simulink model "c00010M_harness"  (R2018a)
settings: Solver=FixedStepAuto  StartTime=0.0  StopTime=300  FixedStep=0.1  RelTol=1e-3
undefined symbols (not defined in the file): A1, hmax, PriorityTank, R1, R2, sigbuilder_block, TempThreshold
(part 1 of 40)
settings Model: Creator=aarrieta  LastModifiedBy=umarkiegi

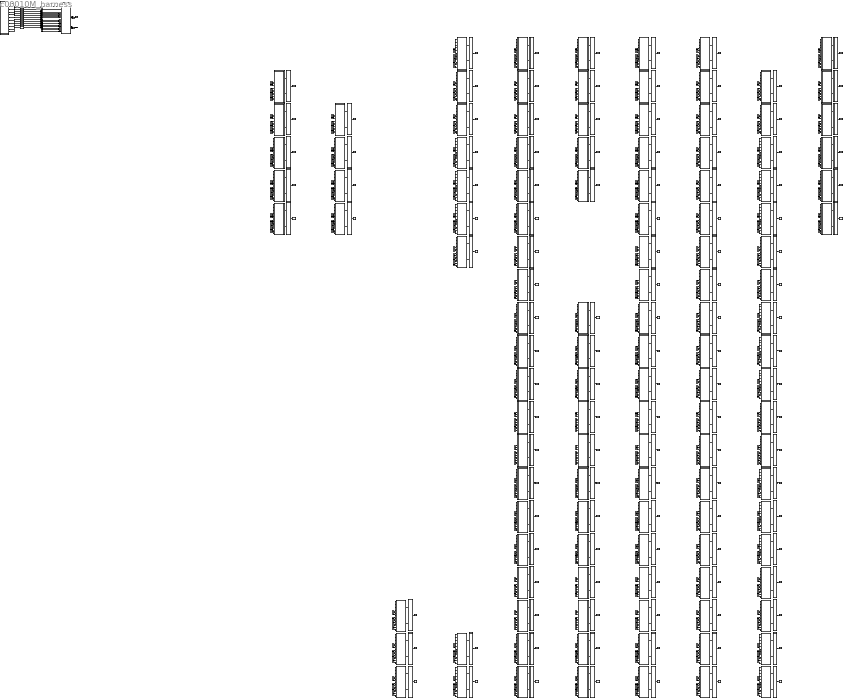
== system c00010M_harness ==
  CPSUT : Subsystem
  Eval117 : Subsystem
  Eval118 : Subsystem
  Eval119 : Subsystem
  Eval120 : Subsystem
  Eval121 : Subsystem
  Eval122 : Subsystem
  Eval123 : Subsystem
  Eval124 : Subsystem
  Eval125 : Subsystem
  Eval126 : Subsystem
  Eval138 : Subsystem
  Eval139 : Subsystem
  Eval140 : Subsystem
  Eval141 : Subsystem
  Eval142 : Subsystem
  Eval143 : Subsystem
  Eval144 : Subsystem
  Eval145 : Subsystem
  Eval146 : Subsystem
  Eval147 : Subsystem
  Eval148 : Subsystem
  Eval149 : Subsystem
  Eval150 : Subsystem
  Eval151 : Subsystem
  Eval152 : Subsystem
  Eval153 : Subsystem
  Eval154 : Subsystem
  Eval155 : Subsystem
  Eval156 : Subsystem
  Eval157 : Subsystem
  Eval158 : Subsystem
  Eval159 : Subsystem
  Eval160 : Subsystem
  Eval161 : Subsystem
  Eval162 : Subsystem
  Eval163 : Subsystem
  Eval164 : Subsystem
  Eval168 : Subsystem
  Eval169 : Subsystem
  Eval170 : Subsystem
  Eval171 : Subsystem
  Eval172 : Subsystem
  Eval173 : Subsystem
  Eval174 : Subsystem
  Eval175 : Subsystem
  Eval176 : Subsystem
  Eval177 : Subsystem
  Eval178 : Subsystem
  Eval179 : Subsystem
  Eval180 : Subsystem
  Eval181 : Subsystem
  Eval182 : Subsystem
  Eval183 : Subsystem
  Eval184 : Subsystem
  Eval185 : Subsystem
  Eval186 : Subsystem
  Eval187 : Subsystem
  Eval188 : Subsystem
  Eval189 : Subsystem
  Eval190 : Subsystem
  Eval191 : Subsystem
  Eval192 : Subsystem
  Eval193 : Subsystem
  Eval194 : Subsystem
  Eval195 : Subsystem
  Eval196 : Subsystem
  Eval197 : Subsystem
  Eval198 : Subsystem
  Eval199 : Subsystem
  Eval200 : Subsystem
  Eval201 : Subsystem
  Eval202 : Subsystem
  Eval203 : Subsystem
  Eval204 : Subsystem
  Eval205 : Subsystem
  Eval206 : Subsystem
  Eval207 : Subsystem
  Eval208 : Subsystem
  Eval209 : Subsystem
  Eval210 : Subsystem
  Eval211 : Subsystem
  Eval212 : Subsystem
  Eval213 : Subsystem
  Eval214 : Subsystem
  Eval215 : Subsystem
  Eval216 : Subsystem
  Eval217 : Subsystem
  Eval218 : Subsystem
  Eval219 : Subsystem
  Eval221 : Subsystem
  Eval222 : Subsystem
  Eval223 : Subsystem
  Eval224 : Subsystem
  Eval225 : Subsystem
  Eval226 : Subsystem
  Eval227 : Subsystem
  Eval228 : Subsystem
  Eval229 : Subsystem
  Eval230 : Subsystem
  Eval231 : Subsystem
  Eval232 : Subsystem
  Eval233 : Subsystem
  Eval234 : Subsystem
  Eval235 : Subsystem
  Eval236 : Subsystem
  Eval237 : Subsystem
  Eval238 : Subsystem
  Eval239 : Subsystem
  Eval240 : Subsystem
  Eval241 : Subsystem
  Eval242 : Subsystem
  Eval243 : Subsystem
  Eval244 : Subsystem
  Eval245 : Subsystem
  Eval61 : Subsystem
  Eval62 : Subsystem
  Eval63 : Subsystem
  Eval64 : Subsystem
  Eval65 : Subsystem
  Eval82 : Subsystem
  Eval83 : Subsystem
  Eval84 : Subsystem
  Eval85 : Subsystem
  Inputs : Subsystem  Tag=STV Subsys  LoadFcn=sigbuilder_block('load');  StartFcn=sigbuilder_block('start');  StopFcn=sigbuilder_block('stop');  ClipboardFcn=sigbuilder_block('clipboard');  mask(Sigbuilder block){tuvar=[0:10]}
      mask init:
      | if ~strcmp(get_param(bdroot(gcb),'SimulationStatus'),'stopped'),tuvar = sigbuilder_block('maskInit'); end
      settings: CopyFcn=sigbuilder_block('copy');  DeleteFcn=sigbuilder_block('delete');  ModelCloseFcn=sigbuilder_block('modelClose');  PreSaveFcn=sigbuilder_block('preSave');  PauseFcn=sigbuilder_block('pause');  ContinueFcn=sigbuilder_block('continue');  NameChangeFcn=sigbuilder_block('namechange');  OpenFcn=sigbuilder_block('open',[276.75 163.5 675.75 486.75 ]);  CloseFcn=sigbuilder_block('close');
      mask Display: plot(0, 0, 100, 100,[2, 2, 32, 32, 2], [68, 8, 8, 68, 68],[32, 2], [38, 38], [32, 19, 2],[53, 60, 44], [32, 17, 17, 2],[16, 16, 31, 31]);txt = getActiveGroup(gcbh);text(2, 100, txt,'verticalAlignment', 'top');
  M062 : Subsystem
  M063 : Subsystem
  M064 : Subsystem
  M065 : Subsystem
  M066 : Subsystem
  M083 : Subsystem
  M084 : Subsystem
  M085 : Subsystem
  M086 : Subsystem
  M118 : Subsystem
  M119 : Subsystem
  M120 : Subsystem
  M121 : Subsystem
  M122 : Subsystem
  M123 : Subsystem
  M124 : Subsystem
  M125 : Subsystem
  M126 : Subsystem
  M127 : Subsystem
  M139 : Subsystem
  M140 : Subsystem
  M141 : Subsystem
  M142 : Subsystem
  M143 : Subsystem
  M144 : Subsystem
  M145 : Subsystem
  M146 : Subsystem
  M147 : Subsystem
  M148 : Subsystem
  M149 : Subsystem
  M150 : Subsystem
  M151 : Subsystem
  M152 : Subsystem
  M153 : Subsystem
  M154 : Subsystem
  M155 : Subsystem
  M156 : Subsystem
  M157 : Subsystem
  M158 : Subsystem
  M159 : Subsystem
  M160 : Subsystem
  M161 : Subsystem
  M162 : Subsystem
  M163 : Subsystem
  M164 : Subsystem
  M165 : Subsystem
  M169 : Subsystem
  M170 : Subsystem
  M171 : Subsystem
  M172 : Subsystem
  M173 : Subsystem
  M174 : Subsystem
  M175 : Subsystem
  M176 : Subsystem
  M177 : Subsystem
  M178 : Subsystem
  M179 : Subsystem
  M180 : Subsystem
  M181 : Subsystem
  M182 : Subsystem
  M183 : Subsystem
  M184 : Subsystem
  M185 : Subsystem
  M186 : Subsystem
  M187 : Subsystem
  M188 : Subsystem
  M189 : Subsystem
  M190 : Subsystem
  M191 : Subsystem
  M192 : Subsystem
  M193 : Subsystem
  M194 : Subsystem
  M195 : Subsystem
  M196 : Subsystem
  M197 : Subsystem
  M198 : Subsystem
  M199 : Subsystem
  M200 : Subsystem
  M201 : Subsystem
  M202 : Subsystem
  M203 : Subsystem
  M204 : Subsystem
  M205 : Subsystem
  M206 : Subsystem
  M207 : Subsystem
  M208 : Subsystem
  M209 : Subsystem
  M210 : Subsystem
  M211 : Subsystem
  M212 : Subsystem
  M213 : Subsystem
  M214 : Subsystem
  M215 : Subsystem
  M216 : Subsystem
  M217 : Subsystem
  M218 : Subsystem
  M219 : Subsystem
  M220 : Subsystem
  M222 : Subsystem
  M223 : Subsystem
  M224 : Subsystem
  M225 : Subsystem
  M226 : Subsystem
  M227 : Subsystem
  M228 : Subsystem
  M229 : Subsystem
  M230 : Subsystem
  M231 : Subsystem
  M232 : Subsystem
  M233 : Subsystem
  M234 : Subsystem
  M235 : Subsystem
  M236 : Subsystem
  M237 : Subsystem
  M238 : Subsystem
  M239 : Subsystem
  M240 : Subsystem
  M241 : Subsystem
  M242 : Subsystem
  M243 : Subsystem
  M244 : Subsystem
  M245 : Subsystem
  M246 : Subsystem
  To Workspace117 : ToWorkspace  VariableName=mutant118  SampleTime=-1
  To Workspace118 : ToWorkspace  VariableName=mutant119  SampleTime=-1
  To Workspace119 : ToWorkspace  VariableName=mutant120  SampleTime=-1
  To Workspace120 : ToWorkspace  VariableName=mutant121  SampleTime=-1
  To Workspace121 : ToWorkspace  VariableName=mutant122  SampleTime=-1
  To Workspace122 : ToWorkspace  VariableName=mutant123  SampleTime=-1
  To Workspace123 : ToWorkspace  VariableName=mutant124  SampleTime=-1
  To Workspace124 : ToWorkspace  VariableName=mutant125  SampleTime=-1
  To Workspace125 : ToWorkspace  VariableName=mutant126  SampleTime=-1
  To Workspace126 : ToWorkspace  VariableName=mutant127  SampleTime=-1
  To Workspace138 : ToWorkspace  VariableName=mutant139  SampleTime=-1
  To Workspace139 : ToWorkspace  VariableName=mutant140  SampleTime=-1
  To Workspace140 : ToWorkspace  VariableName=mutant141  SampleTime=-1
  To Workspace141 : ToWorkspace  VariableName=mutant142  SampleTime=-1
  To Workspace142 : ToWorkspace  VariableName=mutant143  SampleTime=-1
  To Workspace143 : ToWorkspace  VariableName=mutant144  SampleTime=-1
  To Workspace144 : ToWorkspace  VariableName=mutant145  SampleTime=-1
  To Workspace145 : ToWorkspace  VariableName=mutant146  SampleTime=-1
  To Workspace146 : ToWorkspace  VariableName=mutant147  SampleTime=-1
  To Workspace147 : ToWorkspace  VariableName=mutant148  SampleTime=-1
  To Workspace148 : ToWorkspace  VariableName=mutant149  SampleTime=-1
  To Workspace149 : ToWorkspace  VariableName=mutant150  SampleTime=-1
  To Workspace150 : ToWorkspace  VariableName=mutant151  SampleTime=-1
  To Workspace151 : ToWorkspace  VariableName=mutant152  SampleTime=-1
  To Workspace152 : ToWorkspace  VariableName=mutant153  SampleTime=-1
  To Workspace153 : ToWorkspace  VariableName=mutant154  SampleTime=-1
  To Workspace154 : ToWorkspace  VariableName=mutant155  SampleTime=-1
  To Workspace155 : ToWorkspace  VariableName=mutant156  SampleTime=-1
  To Workspace156 : ToWorkspace  VariableName=mutant157  SampleTime=-1
  To Workspace157 : ToWorkspace  VariableName=mutant158  SampleTime=-1
  To Workspace158 : ToWorkspace  VariableName=mutant159  SampleTime=-1
  To Workspace159 : ToWorkspace  VariableName=mutant160  SampleTime=-1
  To Workspace160 : ToWorkspace  VariableName=mutant161  SampleTime=-1
  To Workspace161 : ToWorkspace  VariableName=mutant162  SampleTime=-1
  To Workspace162 : ToWorkspace  VariableName=mutant163  SampleTime=-1
  To Workspace163 : ToWorkspace  VariableName=mutant164  SampleTime=-1
  To Workspace164 : ToWorkspace  VariableName=mutant165  SampleTime=-1
  To Workspace168 : ToWorkspace  VariableName=mutant169  SampleTime=-1
  To Workspace169 : ToWorkspace  VariableName=mutant170  SampleTime=-1
  To Workspace170 : ToWorkspace  VariableName=mutant171  SampleTime=-1
  To Workspace171 : ToWorkspace  VariableName=mutant172  SampleTime=-1
  To Workspace172 : ToWorkspace  VariableName=mutant173  SampleTime=-1
  To Workspace173 : ToWorkspace  VariableName=mutant174  SampleTime=-1
  To Workspace174 : ToWorkspace  VariableName=mutant175  SampleTime=-1
  To Workspace175 : ToWorkspace  VariableName=mutant176  SampleTime=-1
  To Workspace176 : ToWorkspace  VariableName=mutant177  SampleTime=-1
  To Workspace177 : ToWorkspace  VariableName=mutant178  SampleTime=-1
  To Workspace178 : ToWorkspace  VariableName=mutant179  SampleTime=-1
  To Workspace179 : ToWorkspace  VariableName=mutant180  SampleTime=-1
  To Workspace180 : ToWorkspace  VariableName=mutant181  SampleTime=-1
  To Workspace181 : ToWorkspace  VariableName=mutant182  SampleTime=-1
  To Workspace182 : ToWorkspace  VariableName=mutant183  SampleTime=-1
  To Workspace183 : ToWorkspace  VariableName=mutant184  SampleTime=-1
  To Workspace184 : ToWorkspace  VariableName=mutant185  SampleTime=-1
  To Workspace185 : ToWorkspace  VariableName=mutant186  SampleTime=-1
  To Workspace186 : ToWorkspace  VariableName=mutant187  SampleTime=-1
  To Workspace187 : ToWorkspace  VariableName=mutant188  SampleTime=-1
  To Workspace188 : ToWorkspace  VariableName=mutant189  SampleTime=-1
  To Workspace189 : ToWorkspace  VariableName=mutant190  SampleTime=-1
  To Workspace190 : ToWorkspace  VariableName=mutant191  SampleTime=-1
  To Workspace191 : ToWorkspace  VariableName=mutant192  SampleTime=-1
  To Workspace192 : ToWorkspace  VariableName=mutant193  SampleTime=-1
  To Workspace193 : ToWorkspace  VariableName=mutant194  SampleTime=-1
  To Workspace194 : ToWorkspace  VariableName=mutant195  SampleTime=-1
  To Workspace195 : ToWorkspace  VariableName=mutant196  SampleTime=-1
  To Workspace196 : ToWorkspace  VariableName=mutant197  SampleTime=-1
  To Workspace197 : ToWorkspace  VariableName=mutant198  SampleTime=-1
  To Workspace198 : ToWorkspace  VariableName=mutant199  SampleTime=-1
  To Workspace199 : ToWorkspace  VariableName=mutant200  SampleTime=-1
  To Workspace200 : ToWorkspace  VariableName=mutant201  SampleTime=-1
  To Workspace201 : ToWorkspace  VariableName=mutant202  SampleTime=-1
  To Workspace202 : ToWorkspace  VariableName=mutant203  SampleTime=-1
  To Workspace203 : ToWorkspace  VariableName=mutant204  SampleTime=-1
  To Workspace204 : ToWorkspace  VariableName=mutant205  SampleTime=-1
  To Workspace205 : ToWorkspace  VariableName=mutant206  SampleTime=-1
  To Workspace206 : ToWorkspace  VariableName=mutant207  SampleTime=-1
  To Workspace207 : ToWorkspace  VariableName=mutant208  SampleTime=-1
  To Workspace208 : ToWorkspace  VariableName=mutant209  SampleTime=-1
  To Workspace209 : ToWorkspace  VariableName=mutant210  SampleTime=-1
  To Workspace210 : ToWorkspace  VariableName=mutant211  SampleTime=-1
  To Workspace211 : ToWorkspace  VariableName=mutant212  SampleTime=-1
  To Workspace212 : ToWorkspace  VariableName=mutant213  SampleTime=-1
  To Workspace213 : ToWorkspace  VariableName=mutant214  SampleTime=-1
  To Workspace214 : ToWorkspace  VariableName=mutant215  SampleTime=-1
  To Workspace215 : ToWorkspace  VariableName=mutant216  SampleTime=-1
  To Workspace216 : ToWorkspace  VariableName=mutant217  SampleTime=-1
  To Workspace217 : ToWorkspace  VariableName=mutant218  SampleTime=-1
  To Workspace218 : ToWorkspace  VariableName=mutant219  SampleTime=-1
  To Workspace219 : ToWorkspace  VariableName=mutant220  SampleTime=-1
  To Workspace221 : ToWorkspace  VariableName=mutant222  SampleTime=-1
  To Workspace222 : ToWorkspace  VariableName=mutant223  SampleTime=-1
  To Workspace223 : ToWorkspace  VariableName=mutant224  SampleTime=-1
  To Workspace224 : ToWorkspace  VariableName=mutant225  SampleTime=-1
  To Workspace225 : ToWorkspace  VariableName=mutant226  SampleTime=-1
  To Workspace226 : ToWorkspace  VariableName=mutant227  SampleTime=-1
  To Workspace227 : ToWorkspace  VariableName=mutant228  SampleTime=-1
  To Workspace228 : ToWorkspace  VariableName=mutant229  SampleTime=-1
  To Workspace229 : ToWorkspace  VariableName=mutant230  SampleTime=-1
  To Workspace230 : ToWorkspace  VariableName=mutant231  SampleTime=-1
  To Workspace231 : ToWorkspace  VariableName=mutant232  SampleTime=-1
  To Workspace232 : ToWorkspace  VariableName=mutant233  SampleTime=-1
  To Workspace233 : ToWorkspace  VariableName=mutant234  SampleTime=-1
  To Workspace234 : ToWorkspace  VariableName=mutant235  SampleTime=-1
  To Workspace235 : ToWorkspace  VariableName=mutant236  SampleTime=-1
  To Workspace236 : ToWorkspace  VariableName=mutant237  SampleTime=-1
  To Workspace237 : ToWorkspace  VariableName=mutant238  SampleTime=-1
  To Workspace238 : ToWorkspace  VariableName=mutant239  SampleTime=-1
  To Workspace239 : ToWorkspace  VariableName=mutant240  SampleTime=-1
  To Workspace240 : ToWorkspace  VariableName=mutant241  SampleTime=-1
  To Workspace241 : ToWorkspace  VariableName=mutant242  SampleTime=-1
  To Workspace242 : ToWorkspace  VariableName=mutant243  SampleTime=-1
  To Workspace243 : ToWorkspace  VariableName=mutant244  SampleTime=-1
  To Workspace244 : ToWorkspace  VariableName=mutant245  SampleTime=-1
  To Workspace245 : ToWorkspace  VariableName=mutant246  SampleTime=-1
  To Workspace61 : ToWorkspace  VariableName=mutant062  SampleTime=-1
  To Workspace62 : ToWorkspace  VariableName=mutant063  SampleTime=-1
  To Workspace63 : ToWorkspace  VariableName=mutant064  SampleTime=-1
  To Workspace64 : ToWorkspace  VariableName=mutant065  SampleTime=-1
  To Workspace65 : ToWorkspace  VariableName=mutant066  SampleTime=-1
  To Workspace82 : ToWorkspace  VariableName=mutant083  SampleTime=-1
  To Workspace83 : ToWorkspace  VariableName=mutant084  SampleTime=-1
  To Workspace84 : ToWorkspace  VariableName=mutant085  SampleTime=-1
  To Workspace85 : ToWorkspace  VariableName=mutant086  SampleTime=-1
  dtc_CT2 : DataTypeConversion
  dtc_CT3 : DataTypeConversion
  dtc_E2 : DataTypeConversion
  dtc_E3 : DataTypeConversion
  dtc_EB2 : DataTypeConversion
  dtc_EB3 : DataTypeConversion
  dtc_F2 : DataTypeConversion
  dtc_F3 : DataTypeConversion
  dtc_MR3 : DataTypeConversion
  dtc_T2 : DataTypeConversion
  dtc_T3 : DataTypeConversion
  LL2 : Outport
  LL3 : Outport  Port=2
  tag scope: out2=global, out3=global
  wires:
  CPSUT/1(LL2) -> [out2], LL2/1
  CPSUT/2(LL3) -> [out3], LL3/1
  [in7] -> M062/1(CT2)
  [in8] -> M062/2(F2)
  [in9] -> M062/3(E2)
  [in11] -> M062/4(T2)
  [in12] -> M062/5(EB2)
  [in13] -> M062/6(CT3)
  [in14] -> M062/7(F3)
  [in15] -> M062/8(E3)
  [in16] -> M062/9(MR3)
  [in17] -> M062/10(T3)
  [in18] -> M062/11(EB3)
  M062/1(LL2) -> Eval61/1(In2)
  M062/2(LL3) -> Eval61/2(In3)
  Eval61/1(Out1) -> To Workspace61/1
  [in7] -> M063/1(CT2)
  [in8] -> M063/2(F2)
  [in9] -> M063/3(E2)
  [in11] -> M063/4(T2)
  [in12] -> M063/5(EB2)
  [in13] -> M063/6(CT3)
  [in14] -> M063/7(F3)
  [in15] -> M063/8(E3)
  [in16] -> M063/9(MR3)
  [in17] -> M063/10(T3)
  [in18] -> M063/11(EB3)
  M063/1(LL2) -> Eval62/1(In2)
  M063/2(LL3) -> Eval62/2(In3)
  Eval62/1(Out1) -> To Workspace62/1
  [in7] -> M064/1(CT2)
  [in8] -> M064/2(F2)
  [in9] -> M064/3(E2)
  [in11] -> M064/4(T2)
  [in12] -> M064/5(EB2)
  [in13] -> M064/6(CT3)
  [in14] -> M064/7(F3)
  [in15] -> M064/8(E3)
  [in16] -> M064/9(MR3)
  [in17] -> M064/10(T3)
  [in18] -> M064/11(EB3)
  M064/1(LL2) -> Eval63/1(In2)
  M064/2(LL3) -> Eval63/2(In3)
  Eval63/1(Out1) -> To Workspace63/1
  [in7] -> M065/1(CT2)
  [in8] -> M065/2(F2)
  [in9] -> M065/3(E2)
  [in11] -> M065/4(T2)
  [in12] -> M065/5(EB2)
  [in13] -> M065/6(CT3)
  [in14] -> M065/7(F3)
  [in15] -> M065/8(E3)
  [in16] -> M065/9(MR3)
  [in17] -> M065/10(T3)
  [in18] -> M065/11(EB3)
  M065/1(LL2) -> Eval64/1(In2)
  M065/2(LL3) -> Eval64/2(In3)
  Eval64/1(Out1) -> To Workspace64/1
  [in7] -> M066/1(CT2)
  [in8] -> M066/2(F2)
  [in9] -> M066/3(E2)
  [in11] -> M066/4(T2)
  [in12] -> M066/5(EB2)
  [in13] -> M066/6(CT3)
  [in14] -> M066/7(F3)
  [in15] -> M066/8(E3)
  [in16] -> M066/9(MR3)
  [in17] -> M066/10(T3)
  [in18] -> M066/11(EB3)
  M066/1(LL2) -> Eval65/1(In2)
  M066/2(LL3) -> Eval65/2(In3)
  Eval65/1(Out1) -> To Workspace65/1
  [in7] -> M083/1(CT2)
  [in8] -> M083/2(F2)
  [in9] -> M083/3(E2)
  [in11] -> M083/4(T2)
  [in12] -> M083/5(EB2)
  [in13] -> M083/6(CT3)
  [in14] -> M083/7(F3)
  [in15] -> M083/8(E3)
  [in16] -> M083/9(MR3)
  [in17] -> M083/10(T3)
  [in18] -> M083/11(EB3)
  M083/1(LL2) -> Eval82/1(In2)
  M083/2(LL3) -> Eval82/2(In3)
  Eval82/1(Out1) -> To Workspace82/1
  [in7] -> M084/1(CT2)
  [in8] -> M084/2(F2)
  [in9] -> M084/3(E2)
  [in11] -> M084/4(T2)
  [in12] -> M084/5(EB2)
  [in13] -> M084/6(CT3)
  [in14] -> M084/7(F3)
  [in15] -> M084/8(E3)
  [in16] -> M084/9(MR3)
  [in17] -> M084/10(T3)
  [in18] -> M084/11(EB3)
  M084/1(LL2) -> Eval83/1(In2)
  M084/2(LL3) -> Eval83/2(In3)
  Eval83/1(Out1) -> To Workspace83/1
  [in7] -> M085/1(CT2)
  [in8] -> M085/2(F2)
  [in9] -> M085/3(E2)
  [in11] -> M085/4(T2)
  [in12] -> M085/5(EB2)
  [in13] -> M085/6(CT3)
  [in14] -> M085/7(F3)
  [in15] -> M085/8(E3)
  [in16] -> M085/9(MR3)
  [in17] -> M085/10(T3)
  [in18] -> M085/11(EB3)
  M085/1(LL2) -> Eval84/1(In2)
  M085/2(LL3) -> Eval84/2(In3)
  Eval84/1(Out1) -> To Workspace84/1
  [in7] -> M086/1(CT2)
  [in8] -> M086/2(F2)
  [in9] -> M086/3(E2)
  [in11] -> M086/4(T2)
  [in12] -> M086/5(EB2)
  [in13] -> M086/6(CT3)
  [in14] -> M086/7(F3)
  [in15] -> M086/8(E3)
  [in16] -> M086/9(MR3)
  [in17] -> M086/10(T3)
  [in18] -> M086/11(EB3)
  M086/1(LL2) -> Eval85/1(In2)
  M086/2(LL3) -> Eval85/2(In3)
  Eval85/1(Out1) -> To Workspace85/1
  [in7] -> M118/1(CT2)
  [in8] -> M118/2(F2)
  [in9] -> M118/3(E2)
  [in11] -> M118/4(T2)
  [in12] -> M118/5(EB2)
  [in13] -> M118/6(CT3)
  [in14] -> M118/7(F3)
  [in15] -> M118/8(E3)
  [in16] -> M118/9(MR3)
  [in17] -> M118/10(T3)
  [in18] -> M118/11(EB3)
  M118/1(LL2) -> Eval117/1(In2)
  M118/2(LL3) -> Eval117/2(In3)
  Eval117/1(Out1) -> To Workspace117/1
  [in7] -> M119/1(CT2)
  [in8] -> M119/2(F2)
  [in9] -> M119/3(E2)
  [in11] -> M119/4(T2)
  [in12] -> M119/5(EB2)
  [in13] -> M119/6(CT3)
  [in14] -> M119/7(F3)
  [in15] -> M119/8(E3)
  [in16] -> M119/9(MR3)
  [in17] -> M119/10(T3)
  [in18] -> M119/11(EB3)
  M119/1(LL2) -> Eval118/1(In2)
  M119/2(LL3) -> Eval118/2(In3)
  Eval118/1(Out1) -> To Workspace118/1
  [in7] -> M120/1(CT2)
  [in8] -> M120/2(F2)
  [in9] -> M120/3(E2)
  [in11] -> M120/4(T2)
  [in12] -> M120/5(EB2)
  [in13] -> M120/6(CT3)
  [in14] -> M120/7(F3)
  [in15] -> M120/8(E3)
  [in16] -> M120/9(MR3)
  [in17] -> M120/10(T3)
  [in18] -> M120/11(EB3)
  M120/1(LL2) -> Eval119/1(In2)
  M120/2(LL3) -> Eval119/2(In3)
  Eval119/1(Out1) -> To Workspace119/1
  [in7] -> M121/1(CT2)
  [in8] -> M121/2(F2)
  [in9] -> M121/3(E2)
  [in11] -> M121/4(T2)
  [in12] -> M121/5(EB2)
  [in13] -> M121/6(CT3)
  [in14] -> M121/7(F3)
  [in15] -> M121/8(E3)
  [in16] -> M121/9(MR3)
  [in17] -> M121/10(T3)
  [in18] -> M121/11(EB3)
  M121/1(LL2) -> Eval120/1(In2)
  M121/2(LL3) -> Eval120/2(In3)
  Eval120/1(Out1) -> To Workspace120/1
  [in7] -> M122/1(CT2)
  [in8] -> M122/2(F2)
  [in9] -> M122/3(E2)
  [in11] -> M122/4(T2)
  [in12] -> M122/5(EB2)
  [in13] -> M122/6(CT3)
  [in14] -> M122/7(F3)
  [in15] -> M122/8(E3)
  [in16] -> M122/9(MR3)
  [in17] -> M122/10(T3)
  [in18] -> M122/11(EB3)
  M122/1(LL2) -> Eval121/1(In2)
  M122/2(LL3) -> Eval121/2(In3)
  Eval121/1(Out1) -> To Workspace121/1
  [in7] -> M123/1(CT2)
  [in8] -> M123/2(F2)
  [in9] -> M123/3(E2)
  [in11] -> M123/4(T2)
  [in12] -> M123/5(EB2)
  [in13] -> M123/6(CT3)
  [in14] -> M123/7(F3)
  [in15] -> M123/8(E3)
  [in16] -> M123/9(MR3)
  [in17] -> M123/10(T3)
  [in18] -> M123/11(EB3)
  M123/1(LL2) -> Eval122/1(In2)
  M123/2(LL3) -> Eval122/2(In3)
  Eval122/1(Out1) -> To Workspace122/1
  [in7] -> M124/1(CT2)
  [in8] -> M124/2(F2)
  [in9] -> M124/3(E2)
  [in11] -> M124/4(T2)
  [in12] -> M124/5(EB2)
  [in13] -> M124/6(CT3)
  [in14] -> M124/7(F3)
  [in15] -> M124/8(E3)
  [in16] -> M124/9(MR3)
  [in17] -> M124/10(T3)
  [in18] -> M124/11(EB3)
  M124/1(LL2) -> Eval123/1(In2)
  M124/2(LL3) -> Eval123/2(In3)
  Eval123/1(Out1) -> To Workspace123/1
  [in7] -> M125/1(CT2)
  [in8] -> M125/2(F2)
  [in9] -> M125/3(E2)
  [in11] -> M125/4(T2)
  [in12] -> M125/5(EB2)
  [in13] -> M125/6(CT3)
  [in14] -> M125/7(F3)
  [in15] -> M125/8(E3)
  [in16] -> M125/9(MR3)
  [in17] -> M125/10(T3)
  [in18] -> M125/11(EB3)
  M125/1(LL2) -> Eval124/1(In2)
  M125/2(LL3) -> Eval124/2(In3)
  Eval124/1(Out1) -> To Workspace124/1
  [in7] -> M126/1(CT2)
  [in8] -> M126/2(F2)
  [in9] -> M126/3(E2)
  [in11] -> M126/4(T2)
  [in12] -> M126/5(EB2)
  [in13] -> M126/6(CT3)
  [in14] -> M126/7(F3)
  [in15] -> M126/8(E3)
  [in16] -> M126/9(MR3)
  [in17] -> M126/10(T3)
  [in18] -> M126/11(EB3)
  M126/1(LL2) -> Eval125/1(In2)
  M126/2(LL3) -> Eval125/2(In3)
  Eval125/1(Out1) -> To Workspace125/1
  [in7] -> M127/1(CT2)
  [in8] -> M127/2(F2)
  [in9] -> M127/3(E2)
  [in11] -> M127/4(T2)
  [in12] -> M127/5(EB2)
  [in13] -> M127/6(CT3)
  [in14] -> M127/7(F3)
  [in15] -> M127/8(E3)
  [in16] -> M127/9(MR3)
  [in17] -> M127/10(T3)
  [in18] -> M127/11(EB3)
  M127/1(LL2) -> Eval126/1(In2)
  M127/2(LL3) -> Eval126/2(In3)
  Eval126/1(Out1) -> To Workspace126/1
  [in7] -> M139/1(CT2)
  [in8] -> M139/2(F2)
  [in9] -> M139/3(E2)
  [in11] -> M139/4(T2)
  [in12] -> M139/5(EB2)
  [in13] -> M139/6(CT3)
  [in14] -> M139/7(F3)
  [in15] -> M139/8(E3)
  [in16] -> M139/9(MR3)
  [in17] -> M139/10(T3)
  [in18] -> M139/11(EB3)
  M139/1(LL2) -> Eval138/1(In2)
  M139/2(LL3) -> Eval138/2(In3)
  Eval138/1(Out1) -> To Workspace138/1
  [in7] -> M140/1(CT2)
  [in8] -> M140/2(F2)
  [in9] -> M140/3(E2)
  [in11] -> M140/4(T2)
  [in12] -> M140/5(EB2)
  [in13] -> M140/6(CT3)
  [in14] -> M140/7(F3)
  [in15] -> M140/8(E3)
  [in16] -> M140/9(MR3)
  [in17] -> M140/10(T3)
  [in18] -> M140/11(EB3)
  M140/1(LL2) -> Eval139/1(In2)
  M140/2(LL3) -> Eval139/2(In3)
  Eval139/1(Out1) -> To Workspace139/1
  [in7] -> M141/1(CT2)
  [in8] -> M141/2(F2)
  [in9] -> M141/3(E2)
  [in11] -> M141/4(T2)
  [in12] -> M141/5(EB2)
  [in13] -> M141/6(CT3)
  [in14] -> M141/7(F3)
  [in15] -> M141/8(E3)
  [in16] -> M141/9(MR3)
  [in17] -> M141/10(T3)
  [in18] -> M141/11(EB3)
  M141/1(LL2) -> Eval140/1(In2)
  M141/2(LL3) -> Eval140/2(In3)
  Eval140/1(Out1) -> To Workspace140/1
  [in7] -> M142/1(CT2)
  [in8] -> M142/2(F2)
  [in9] -> M142/3(E2)
  [in11] -> M142/4(T2)
  [in12] -> M142/5(EB2)
  [in13] -> M142/6(CT3)
  [in14] -> M142/7(F3)
  [in15] -> M142/8(E3)
  [in16] -> M142/9(MR3)
  [in17] -> M142/10(T3)
  [in18] -> M142/11(EB3)
  M142/1(LL2) -> Eval141/1(In2)
  M142/2(LL3) -> Eval141/2(In3)
  Eval141/1(Out1) -> To Workspace141/1
  [in7] -> M143/1(CT2)
  [in8] -> M143/2(F2)
  [in9] -> M143/3(E2)
  [in11] -> M143/4(T2)
  [in12] -> M143/5(EB2)
  [in13] -> M143/6(CT3)
  [in14] -> M143/7(F3)
  [in15] -> M143/8(E3)
  [in16] -> M143/9(MR3)
  [in17] -> M143/10(T3)
  [in18] -> M143/11(EB3)
  M143/1(LL2) -> Eval142/1(In2)
  M143/2(LL3) -> Eval142/2(In3)
  Eval142/1(Out1) -> To Workspace142/1
  [in7] -> M144/1(CT2)
  [in8] -> M144/2(F2)
  [in9] -> M144/3(E2)
  [in11] -> M144/4(T2)
  [in12] -> M144/5(EB2)
  [in13] -> M144/6(CT3)
  [in14] -> M144/7(F3)
  [in15] -> M144/8(E3)
  [in16] -> M144/9(MR3)
  [in17] -> M144/10(T3)
  [in18] -> M144/11(EB3)
  M144/1(LL2) -> Eval143/1(In2)
  M144/2(LL3) -> Eval143/2(In3)
  Eval143/1(Out1) -> To Workspace143/1
  [in7] -> M145/1(CT2)
  [in8] -> M145/2(F2)
  [in9] -> M145/3(E2)
  [in11] -> M145/4(T2)
  [in12] -> M145/5(EB2)
  [in13] -> M145/6(CT3)
  [in14] -> M145/7(F3)
  [in15] -> M145/8(E3)
  [in16] -> M145/9(MR3)
  [in17] -> M145/10(T3)
  [in18] -> M145/11(EB3)
  M145/1(LL2) -> Eval144/1(In2)
  M145/2(LL3) -> Eval144/2(In3)
  Eval144/1(Out1) -> To Workspace144/1
  [in7] -> M146/1(CT2)
  [in8] -> M146/2(F2)
  [in9] -> M146/3(E2)
  [in11] -> M146/4(T2)
  [in12] -> M146/5(EB2)
  [in13] -> M146/6(CT3)
  [in14] -> M146/7(F3)
  [in15] -> M146/8(E3)
  [in16] -> M146/9(MR3)
  [in17] -> M146/10(T3)
  [in18] -> M146/11(EB3)
  M146/1(LL2) -> Eval145/1(In2)
  M146/2(LL3) -> Eval145/2(In3)
  Eval145/1(Out1) -> To Workspace145/1
  [in7] -> M147/1(CT2)
  [in8] -> M147/2(F2)
  [in9] -> M147/3(E2)
  [in11] -> M147/4(T2)
  [in12] -> M147/5(EB2)
  [in13] -> M147/6(CT3)
  [in14] -> M147/7(F3)
  [in15] -> M147/8(E3)
  [in16] -> M147/9(MR3)
  [in17] -> M147/10(T3)
  [in18] -> M147/11(EB3)
  M147/1(LL2) -> Eval146/1(In2)
  M147/2(LL3) -> Eval146/2(In3)
  Eval146/1(Out1) -> To Workspace146/1
  [in7] -> M148/1(CT2)
  [in8] -> M148/2(F2)
  [in9] -> M148/3(E2)
  [in11] -> M148/4(T2)
  [in12] -> M148/5(EB2)
  [in13] -> M148/6(CT3)
  [in14] -> M148/7(F3)
  [in15] -> M148/8(E3)
  [in16] -> M148/9(MR3)
  [in17] -> M148/10(T3)
  [in18] -> M148/11(EB3)
  M148/1(LL2) -> Eval147/1(In2)
  M148/2(LL3) -> Eval147/2(In3)
  Eval147/1(Out1) -> To Workspace147/1
  [in7] -> M149/1(CT2)
  [in8] -> M149/2(F2)
  [in9] -> M149/3(E2)
  [in11] -> M149/4(T2)
  [in12] -> M149/5(EB2)
  [in13] -> M149/6(CT3)
  [in14] -> M149/7(F3)
  [in15] -> M149/8(E3)
  [in16] -> M149/9(MR3)
  [in17] -> M149/10(T3)
  [in18] -> M149/11(EB3)
  M149/1(LL2) -> Eval148/1(In2)
  M149/2(LL3) -> Eval148/2(In3)
  Eval148/1(Out1) -> To Workspace148/1
  [in7] -> M150/1(CT2)
  [in8] -> M150/2(F2)
  [in9] -> M150/3(E2)
  [in11] -> M150/4(T2)
  [in12] -> M150/5(EB2)
  [in13] -> M150/6(CT3)
  [in14] -> M150/7(F3)
  [in15] -> M150/8(E3)
  [in16] -> M150/9(MR3)
  [in17] -> M150/10(T3)
  [in18] -> M150/11(EB3)
  M150/1(LL2) -> Eval149/1(In2)
  M150/2(LL3) -> Eval149/2(In3)
  Eval149/1(Out1) -> To Workspace149/1
  [in7] -> M151/1(CT2)
  [in8] -> M151/2(F2)
  [in9] -> M151/3(E2)
  [in11] -> M151/4(T2)
  [in12] -> M151/5(EB2)
  [in13] -> M151/6(CT3)
  [in14] -> M151/7(F3)
  [in15] -> M151/8(E3)
  [in16] -> M151/9(MR3)
  [in17] -> M151/10(T3)
  [in18] -> M151/11(EB3)
  M151/1(LL2) -> Eval150/1(In2)
  M151/2(LL3) -> Eval150/2(In3)
  Eval150/1(Out1) -> To Workspace150/1
  [in7] -> M152/1(CT2)
  [in8] -> M152/2(F2)
  [in9] -> M152/3(E2)
  [in11] -> M152/4(T2)
  [in12] -> M152/5(EB2)
  [in13] -> M152/6(CT3)
  [in14] -> M152/7(F3)
  [in15] -> M152/8(E3)
  [in16] -> M152/9(MR3)
  [in17] -> M152/10(T3)
  [in18] -> M152/11(EB3)
  M152/1(LL2) -> Eval151/1(In2)
  M152/2(LL3) -> Eval151/2(In3)
  Eval151/1(Out1) -> To Workspace151/1
  [in7] -> M153/1(CT2)
  [in8] -> M153/2(F2)
  [in9] -> M153/3(E2)
  [in11] -> M153/4(T2)
  [in12] -> M153/5(EB2)
  [in13] -> M153/6(CT3)
  [in14] -> M153/7(F3)
  [in15] -> M153/8(E3)
  [in16] -> M153/9(MR3)
  [in17] -> M153/10(T3)
  [in18] -> M153/11(EB3)
  M153/1(LL2) -> Eval152/1(In2)
  M153/2(LL3) -> Eval152/2(In3)
  Eval152/1(Out1) -> To Workspace152/1
  [in7] -> M154/1(CT2)
  [in8] -> M154/2(F2)
  [in9] -> M154/3(E2)
  [in11] -> M154/4(T2)
  [in12] -> M154/5(EB2)
  [in13] -> M154/6(CT3)
  [in14] -> M154/7(F3)
  [in15] -> M154/8(E3)
  [in16] -> M154/9(MR3)
  [in17] -> M154/10(T3)
  [in18] -> M154/11(EB3)
  M154/1(LL2) -> Eval153/1(In2)
  M154/2(LL3) -> Eval153/2(In3)
  Eval153/1(Out1) -> To Workspace153/1
  [in7] -> M155/1(CT2)
  [in8] -> M155/2(F2)
  [in9] -> M155/3(E2)
  [in11] -> M155/4(T2)
  [in12] -> M155/5(EB2)
  [in13] -> M155/6(CT3)
  [in14] -> M155/7(F3)
  [in15] -> M155/8(E3)
  [in16] -> M155/9(MR3)
  [in17] -> M155/10(T3)
  [in18] -> M155/11(EB3)
  M155/1(LL2) -> Eval154/1(In2)
  M155/2(LL3) -> Eval154/2(In3)
  Eval154/1(Out1) -> To Workspace154/1
  [in7] -> M156/1(CT2)
  [in8] -> M156/2(F2)
  [in9] -> M156/3(E2)
  [in11] -> M156/4(T2)
  [in12] -> M156/5(EB2)
  [in13] -> M156/6(CT3)
  [in14] -> M156/7(F3)
  [in15] -> M156/8(E3)
  [in16] -> M156/9(MR3)
  [in17] -> M156/10(T3)
  [in18] -> M156/11(EB3)
  M156/1(LL2) -> Eval155/1(In2)
  M156/2(LL3) -> Eval155/2(In3)
  Eval155/1(Out1) -> To Workspace155/1
  [in7] -> M157/1(CT2)
  [in8] -> M157/2(F2)
  [in9] -> M157/3(E2)
  [in11] -> M157/4(T2)
  [in12] -> M157/5(EB2)
  [in13] -> M157/6(CT3)
  [in14] -> M157/7(F3)
  [in15] -> M157/8(E3)
  [in16] -> M157/9(MR3)
  [in17] -> M157/10(T3)
  [in18] -> M157/11(EB3)
  M157/1(LL2) -> Eval156/1(In2)
  M157/2(LL3) -> Eval156/2(In3)
  Eval156/1(Out1) -> To Workspace156/1
  [in7] -> M158/1(CT2)
  [in8] -> M158/2(F2)
  [in9] -> M158/3(E2)
  [in11] -> M158/4(T2)
  [in12] -> M158/5(EB2)
  [in13] -> M158/6(CT3)
  [in14] -> M158/7(F3)
  [in15] -> M158/8(E3)
  [in16] -> M158/9(MR3)
  [in17] -> M158/10(T3)
  [in18] -> M158/11(EB3)
  M158/1(LL2) -> Eval157/1(In2)
  M158/2(LL3) -> Eval157/2(In3)
  Eval157/1(Out1) -> To Workspace157/1
  [in7] -> M159/1(CT2)
  [in8] -> M159/2(F2)
  [in9] -> M159/3(E2)
  [in11] -> M159/4(T2)
  [in12] -> M159/5(EB2)
  [in13] -> M159/6(CT3)
  [in14] -> M159/7(F3)
  [in15] -> M159/8(E3)
  [in16] -> M159/9(MR3)
  [in17] -> M159/10(T3)
  [in18] -> M159/11(EB3)
  M159/1(LL2) -> Eval158/1(In2)
  M159/2(LL3) -> Eval158/2(In3)
  Eval158/1(Out1) -> To Workspace158/1
  [in7] -> M160/1(CT2)
  [in8] -> M160/2(F2)
  [in9] -> M160/3(E2)
  [in11] -> M160/4(T2)
  [in12] -> M160/5(EB2)
  [in13] -> M160/6(CT3)
  [in14] -> M160/7(F3)
  [in15] -> M160/8(E3)
  [in16] -> M160/9(MR3)
  [in17] -> M160/10(T3)
  [in18] -> M160/11(EB3)
  M160/1(LL2) -> Eval159/1(In2)
  M160/2(LL3) -> Eval159/2(In3)
  Eval159/1(Out1) -> To Workspace159/1
  [in7] -> M161/1(CT2)
  [in8] -> M161/2(F2)
  [in9] -> M161/3(E2)
  [in11] -> M161/4(T2)
  [in12] -> M161/5(EB2)
  [in13] -> M161/6(CT3)
  [in14] -> M161/7(F3)
  [in15] -> M161/8(E3)
  [in16] -> M161/9(MR3)
  [in17] -> M161/10(T3)
  [in18] -> M161/11(EB3)
  M161/1(LL2) -> Eval160/1(In2)
  M161/2(LL3) -> Eval160/2(In3)
  Eval160/1(Out1) -> To Workspace160/1
  [in7] -> M162/1(CT2)
  [in8] -> M162/2(F2)
  [in9] -> M162/3(E2)
  [in11] -> M162/4(T2)
  [in12] -> M162/5(EB2)
  [in13] -> M162/6(CT3)
  [in14] -> M162/7(F3)
  [in15] -> M162/8(E3)
  [in16] -> M162/9(MR3)
  [in17] -> M162/10(T3)
  [in18] -> M162/11(EB3)
  M162/1(LL2) -> Eval161/1(In2)
  M162/2(LL3) -> Eval161/2(In3)
  Eval161/1(Out1) -> To Workspace161/1
  [in7] -> M163/1(CT2)
  [in8] -> M163/2(F2)
  [in9] -> M163/3(E2)
  [in11] -> M163/4(T2)
  [in12] -> M163/5(EB2)
  [in13] -> M163/6(CT3)
  [in14] -> M163/7(F3)
  [in15] -> M163/8(E3)
  [in16] -> M163/9(MR3)
  [in17] -> M163/10(T3)
  [in18] -> M163/11(EB3)
  M163/1(LL2) -> Eval162/1(In2)
  M163/2(LL3) -> Eval162/2(In3)
  Eval162/1(Out1) -> To Workspace162/1
  [in7] -> M164/1(CT2)
  [in8] -> M164/2(F2)
  [in9] -> M164/3(E2)
  [in11] -> M164/4(T2)
  [in12] -> M164/5(EB2)
  [in13] -> M164/6(CT3)
  [in14] -> M164/7(F3)
  [in15] -> M164/8(E3)
  [in16] -> M164/9(MR3)
  [in17] -> M164/10(T3)
  [in18] -> M164/11(EB3)
  M164/1(LL2) -> Eval163/1(In2)
  M164/2(LL3) -> Eval163/2(In3)
  Eval163/1(Out1) -> To Workspace163/1
  [in7] -> M165/1(CT2)
  [in8] -> M165/2(F2)
  [in9] -> M165/3(E2)
  [in11] -> M165/4(T2)
  [in12] -> M165/5(EB2)
  [in13] -> M165/6(CT3)
  [in14] -> M165/7(F3)
  [in15] -> M165/8(E3)
  [in16] -> M165/9(MR3)
  [in17] -> M165/10(T3)
  [in18] -> M165/11(EB3)
  M165/1(LL2) -> Eval164/1(In2)
  M165/2(LL3) -> Eval164/2(In3)
  Eval164/1(Out1) -> To Workspace164/1
  [in7] -> M169/1(CT2)
  [in8] -> M169/2(F2)
  [in9] -> M169/3(E2)
  [in11] -> M169/4(T2)
  [in12] -> M169/5(EB2)
  [in13] -> M169/6(CT3)
  [in14] -> M169/7(F3)
  [in15] -> M169/8(E3)
  [in16] -> M169/9(MR3)
  [in17] -> M169/10(T3)
  [in18] -> M169/11(EB3)
  M169/1(LL2) -> Eval168/1(In2)
  M169/2(LL3) -> Eval168/2(In3)
  Eval168/1(Out1) -> To Workspace168/1
  [in7] -> M170/1(CT2)
  [in8] -> M170/2(F2)
  [in9] -> M170/3(E2)
  [in11] -> M170/4(T2)
  [in12] -> M170/5(EB2)
  [in13] -> M170/6(CT3)
  [in14] -> M170/7(F3)
  [in15] -> M170/8(E3)
  [in16] -> M170/9(MR3)
  [in17] -> M170/10(T3)
  [in18] -> M170/11(EB3)
  M170/1(LL2) -> Eval169/1(In2)
  M170/2(LL3) -> Eval169/2(In3)
  Eval169/1(Out1) -> To Workspace169/1
  [in7] -> M171/1(CT2)
  [in8] -> M171/2(F2)
  [in9] -> M171/3(E2)
  [in11] -> M171/4(T2)
  [in12] -> M171/5(EB2)
  [in13] -> M171/6(CT3)
  [in14] -> M171/7(F3)
  [in15] -> M171/8(E3)
  [in16] -> M171/9(MR3)
  [in17] -> M171/10(T3)
  [in18] -> M171/11(EB3)
  M171/1(LL2) -> Eval170/1(In2)
  M171/2(LL3) -> Eval170/2(In3)
  Eval170/1(Out1) -> To Workspace170/1
  [in7] -> M172/1(CT2)
  [in8] -> M172/2(F2)
  [in9] -> M172/3(E2)
  [in11] -> M172/4(T2)
  [in12] -> M172/5(EB2)
  [in13] -> M172/6(CT3)
  [in14] -> M172/7(F3)
  [in15] -> M172/8(E3)
  [in16] -> M172/9(MR3)
  [in17] -> M172/10(T3)
  [in18] -> M172/11(EB3)
  M172/1(LL2) -> Eval171/1(In2)
  M172/2(LL3) -> Eval171/2(In3)
  Eval171/1(Out1) -> To Workspace171/1
  [in7] -> M173/1(CT2)
  [in8] -> M173/2(F2)
  [in9] -> M173/3(E2)
  [in11] -> M173/4(T2)
  [in12] -> M173/5(EB2)
  [in13] -> M173/6(CT3)
  [in14] -> M173/7(F3)
  [in15] -> M173/8(E3)
  [in16] -> M173/9(MR3)
  [in17] -> M173/10(T3)
  [in18] -> M173/11(EB3)
  M173/1(LL2) -> Eval172/1(In2)
  M173/2(LL3) -> Eval172/2(In3)
  Eval172/1(Out1) -> To Workspace172/1
  [in7] -> M174/1(CT2)
  [in8] -> M174/2(F2)
  [in9] -> M174/3(E2)
  [in11] -> M174/4(T2)
  [in12] -> M174/5(EB2)
  [in13] -> M174/6(CT3)
  [in14] -> M174/7(F3)
  [in15] -> M174/8(E3)
  [in16] -> M174/9(MR3)
  [in17] -> M174/10(T3)
  [in18] -> M174/11(EB3)
  M174/1(LL2) -> Eval173/1(In2)
  M174/2(LL3) -> Eval173/2(In3)
  Eval173/1(Out1) -> To Workspace173/1
  [in7] -> M175/1(CT2)
  [in8] -> M175/2(F2)
  [in9] -> M175/3(E2)
  [in11] -> M175/4(T2)
  [in12] -> M175/5(EB2)
  [in13] -> M175/6(CT3)
  [in14] -> M175/7(F3)
  [in15] -> M175/8(E3)
  [in16] -> M175/9(MR3)
  [in17] -> M175/10(T3)
  [in18] -> M175/11(EB3)
  M175/1(LL2) -> Eval174/1(In2)
  M175/2(LL3) -> Eval174/2(In3)
  Eval174/1(Out1) -> To Workspace174/1
  [in7] -> M176/1(CT2)
  [in8] -> M176/2(F2)
  [in9] -> M176/3(E2)
  [in11] -> M176/4(T2)
  [in12] -> M176/5(EB2)
  [in13] -> M176/6(CT3)
  [in14] -> M176/7(F3)
  [in15] -> M176/8(E3)
  [in16] -> M176/9(MR3)
  [in17] -> M176/10(T3)
  [in18] -> M176/11(EB3)
  M176/1(LL2) -> Eval175/1(In2)
  M176/2(LL3) -> Eval175/2(In3)
  Eval175/1(Out1) -> To Workspace175/1
  [in7] -> M177/1(CT2)
  [in8] -> M177/2(F2)
  [in9] -> M177/3(E2)
  [in11] -> M177/4(T2)
  [in12] -> M177/5(EB2)
  [in13] -> M177/6(CT3)
  [in14] -> M177/7(F3)
  [in15] -> M177/8(E3)
  [in16] -> M177/9(MR3)
  [in17] -> M177/10(T3)
  [in18] -> M177/11(EB3)
  M177/1(LL2) -> Eval176/1(In2)
  M177/2(LL3) -> Eval176/2(In3)
  Eval176/1(Out1) -> To Workspace176/1
  [in7] -> M178/1(CT2)
  [in8] -> M178/2(F2)
  [in9] -> M178/3(E2)
  [in11] -> M178/4(T2)
  [in12] -> M178/5(EB2)
  [in13] -> M178/6(CT3)
  [in14] -> M178/7(F3)
  [in15] -> M178/8(E3)
  [in16] -> M178/9(MR3)
  [in17] -> M178/10(T3)
  [in18] -> M178/11(EB3)
  M178/1(LL2) -> Eval177/1(In2)
  M178/2(LL3) -> Eval177/2(In3)
  Eval177/1(Out1) -> To Workspace177/1
  [in7] -> M179/1(CT2)
  [in8] -> M179/2(F2)
  [in9] -> M179/3(E2)
  [in11] -> M179/4(T2)
  [in12] -> M179/5(EB2)
  [in13] -> M179/6(CT3)
  [in14] -> M179/7(F3)
  [in15] -> M179/8(E3)
  [in16] -> M179/9(MR3)
  [in17] -> M179/10(T3)
  [in18] -> M179/11(EB3)
  M179/1(LL2) -> Eval178/1(In2)
  M179/2(LL3) -> Eval178/2(In3)
  Eval178/1(Out1) -> To Workspace178/1
  [in7] -> M180/1(CT2)
  [in8] -> M180/2(F2)
  [in9] -> M180/3(E2)
  [in11] -> M180/4(T2)
  [in12] -> M180/5(EB2)
  [in13] -> M180/6(CT3)
  [in14] -> M180/7(F3)
  [in15] -> M180/8(E3)
  [in16] -> M180/9(MR3)
  [in17] -> M180/10(T3)
  [in18] -> M180/11(EB3)
  M180/1(LL2) -> Eval179/1(In2)
  M180/2(LL3) -> Eval179/2(In3)
  Eval179/1(Out1) -> To Workspace179/1
  [in7] -> M181/1(CT2)
  [in8] -> M181/2(F2)
  [in9] -> M181/3(E2)
  [in11] -> M181/4(T2)
  [in12] -> M181/5(EB2)
  [in13] -> M181/6(CT3)
  [in14] -> M181/7(F3)
  [in15] -> M181/8(E3)
  [in16] -> M181/9(MR3)
  [in17] -> M181/10(T3)
  [in18] -> M181/11(EB3)
  M181/1(LL2) -> Eval180/1(In2)
  M181/2(LL3) -> Eval180/2(In3)
  Eval180/1(Out1) -> To Workspace180/1
  [in7] -> M182/1(CT2)
  [in8] -> M182/2(F2)
  [in9] -> M182/3(E2)
  [in11] -> M182/4(T2)
  [in12] -> M182/5(EB2)
  [in13] -> M182/6(CT3)
  [in14] -> M182/7(F3)
  [in15] -> M182/8(E3)
  [in16] -> M182/9(MR3)
  [in17] -> M182/10(T3)
  [in18] -> M182/11(EB3)
  M182/1(LL2) -> Eval181/1(In2)
  M182/2(LL3) -> Eval181/2(In3)
  Eval181/1(Out1) -> To Workspace181/1
  [in7] -> M183/1(CT2)
  [in8] -> M183/2(F2)
  [in9] -> M183/3(E2)
  [in11] -> M183/4(T2)
  [in12] -> M183/5(EB2)
  [in13] -> M183/6(CT3)
  [in14] -> M183/7(F3)
  [in15] -> M183/8(E3)
  [in16] -> M183/9(MR3)
  [in17] -> M183/10(T3)
  [in18] -> M183/11(EB3)
  M183/1(LL2) -> Eval182/1(In2)
  M183/2(LL3) -> Eval182/2(In3)
  Eval182/1(Out1) -> To Workspace182/1
  [in7] -> M184/1(CT2)
  [in8] -> M184/2(F2)
  [in9] -> M184/3(E2)
  [in11] -> M184/4(T2)
  [in12] -> M184/5(EB2)
  [in13] -> M184/6(CT3)
  [in14] -> M184/7(F3)
  [in15] -> M184/8(E3)
  [in16] -> M184/9(MR3)
  [in17] -> M184/10(T3)
  [in18] -> M184/11(EB3)
  M184/1(LL2) -> Eval183/1(In2)
  M184/2(LL3) -> Eval183/2(In3)
  Eval183/1(Out1) -> To Workspace183/1
  [in7] -> M185/1(CT2)
  [in8] -> M185/2(F2)
  [in9] -> M185/3(E2)
  [in11] -> M185/4(T2)
  [in12] -> M185/5(EB2)
  [in13] -> M185/6(CT3)
  [in14] -> M185/7(F3)
  [in15] -> M185/8(E3)
  [in16] -> M185/9(MR3)
  [in17] -> M185/10(T3)
  [in18] -> M185/11(EB3)
  M185/1(LL2) -> Eval184/1(In2)
  M185/2(LL3) -> Eval184/2(In3)
  Eval184/1(Out1) -> To Workspace184/1
  [in7] -> M186/1(CT2)
  [in8] -> M186/2(F2)
  [in9] -> M186/3(E2)
  [in11] -> M186/4(T2)
  [in12] -> M186/5(EB2)
  [in13] -> M186/6(CT3)
  [in14] -> M186/7(F3)
  [in15] -> M186/8(E3)
  [in16] -> M186/9(MR3)
  [in17] -> M186/10(T3)
  [in18] -> M186/11(EB3)
  M186/1(LL2) -> Eval185/1(In2)
  M186/2(LL3) -> Eval185/2(In3)
  Eval185/1(Out1) -> To Workspace185/1
  [in7] -> M187/1(CT2)
  [in8] -> M187/2(F2)
  [in9] -> M187/3(E2)
  [in11] -> M187/4(T2)
  [in12] -> M187/5(EB2)
  [in13] -> M187/6(CT3)
  [in14] -> M187/7(F3)
  [in15] -> M187/8(E3)
  [in16] -> M187/9(MR3)
  [in17] -> M187/10(T3)
  [in18] -> M187/11(EB3)
  M187/1(LL2) -> Eval186/1(In2)
  M187/2(LL3) -> Eval186/2(In3)
  Eval186/1(Out1) -> To Workspace186/1
  [in7] -> M188/1(CT2)
  [in8] -> M188/2(F2)
  [in9] -> M188/3(E2)
  [in11] -> M188/4(T2)
  [in12] -> M188/5(EB2)
  [in13] -> M188/6(CT3)
  [in14] -> M188/7(F3)
  [in15] -> M188/8(E3)
  [in16] -> M188/9(MR3)
  [in17] -> M188/10(T3)
  [in18] -> M188/11(EB3)
  M188/1(LL2) -> Eval187/1(In2)
  M188/2(LL3) -> Eval187/2(In3)
  Eval187/1(Out1) -> To Workspace187/1
  [in7] -> M189/1(CT2)
  [in8] -> M189/2(F2)
  [in9] -> M189/3(E2)
  [in11] -> M189/4(T2)
  [in12] -> M189/5(EB2)
  [in13] -> M189/6(CT3)
  [in14] -> M189/7(F3)
  [in15] -> M189/8(E3)
  [in16] -> M189/9(MR3)
  [in17] -> M189/10(T3)
  [in18] -> M189/11(EB3)
  M189/1(LL2) -> Eval188/1(In2)
  M189/2(LL3) -> Eval188/2(In3)
  Eval188/1(Out1) -> To Workspace188/1
  [in7] -> M190/1(CT2)
  [in8] -> M190/2(F2)
  [in9] -> M190/3(E2)
  [in11] -> M190/4(T2)
  [in12] -> M190/5(EB2)
  [in13] -> M190/6(CT3)
  [in14] -> M190/7(F3)
  [in15] -> M190/8(E3)
  [in16] -> M190/9(MR3)
  [in17] -> M190/10(T3)
  [in18] -> M190/11(EB3)
  M190/1(LL2) -> Eval189/1(In2)
  M190/2(LL3) -> Eval189/2(In3)
  Eval189/1(Out1) -> To Workspace189/1
  [in7] -> M191/1(CT2)
  [in8] -> M191/2(F2)
  [in9] -> M191/3(E2)
  [in11] -> M191/4(T2)
  [in12] -> M191/5(EB2)
  [in13] -> M191/6(CT3)
  [in14] -> M191/7(F3)
  [in15] -> M191/8(E3)
  [in16] -> M191/9(MR3)
  [in17] -> M191/10(T3)
  [in18] -> M191/11(EB3)
  M191/1(LL2) -> Eval190/1(In2)
  M191/2(LL3) -> Eval190/2(In3)
  Eval190/1(Out1) -> To Workspace190/1
  [in7] -> M192/1(CT2)
  [in8] -> M192/2(F2)
  [in9] -> M192/3(E2)
  [in11] -> M192/4(T2)
  [in12] -> M192/5(EB2)
  [in13] -> M192/6(CT3)
  [in14] -> M192/7(F3)
  [in15] -> M192/8(E3)
  [in16] -> M192/9(MR3)
  [in17] -> M192/10(T3)
  [in18] -> M192/11(EB3)
  M192/1(LL2) -> Eval191/1(In2)
  M192/2(LL3) -> Eval191/2(In3)
  Eval191/1(Out1) -> To Workspace191/1
  [in7] -> M193/1(CT2)
  [in8] -> M193/2(F2)
  [in9] -> M193/3(E2)
  [in11] -> M193/4(T2)
  [in12] -> M193/5(EB2)
  [in13] -> M193/6(CT3)
  [in14] -> M193/7(F3)
  [in15] -> M193/8(E3)
  [in16] -> M193/9(MR3)
  [in17] -> M193/10(T3)
  [in18] -> M193/11(EB3)
  M193/1(LL2) -> Eval192/1(In2)
  M193/2(LL3) -> Eval192/2(In3)
  Eval192/1(Out1) -> To Workspace192/1
  [in7] -> M194/1(CT2)
  [in8] -> M194/2(F2)
  [in9] -> M194/3(E2)
  [in11] -> M194/4(T2)
  [in12] -> M194/5(EB2)
  [in13] -> M194/6(CT3)
  [in14] -> M194/7(F3)
  [in15] -> M194/8(E3)
  [in16] -> M194/9(MR3)
  [in17] -> M194/10(T3)
  [in18] -> M194/11(EB3)
  M194/1(LL2) -> Eval193/1(In2)
  M194/2(LL3) -> Eval193/2(In3)
  Eval193/1(Out1) -> To Workspace193/1
  [in7] -> M195/1(CT2)
  [in8] -> M195/2(F2)
  [in9] -> M195/3(E2)
  [in11] -> M195/4(T2)
  [in12] -> M195/5(EB2)
  [in13] -> M195/6(CT3)
  [in14] -> M195/7(F3)
  [in15] -> M195/8(E3)
  [in16] -> M195/9(MR3)
  [in17] -> M195/10(T3)
  [in18] -> M195/11(EB3)
  M195/1(LL2) -> Eval194/1(In2)
  M195/2(LL3) -> Eval194/2(In3)
  Eval194/1(Out1) -> To Workspace194/1
  [in7] -> M196/1(CT2)
  [in8] -> M196/2(F2)
  [in9] -> M196/3(E2)
  [in11] -> M196/4(T2)
  [in12] -> M196/5(EB2)
  [in13] -> M196/6(CT3)
  [in14] -> M196/7(F3)
  [in15] -> M196/8(E3)
  [in16] -> M196/9(MR3)
  [in17] -> M196/10(T3)
  [in18] -> M196/11(EB3)
  M196/1(LL2) -> Eval195/1(In2)
  M196/2(LL3) -> Eval195/2(In3)
  Eval195/1(Out1) -> To Workspace195/1
  [in7] -> M197/1(CT2)
  [in8] -> M197/2(F2)
  [in9] -> M197/3(E2)
  [in11] -> M197/4(T2)
  [in12] -> M197/5(EB2)
  [in13] -> M197/6(CT3)
  [in14] -> M197/7(F3)
  [in15] -> M197/8(E3)
  [in16] -> M197/9(MR3)
  [in17] -> M197/10(T3)
  [in18] -> M197/11(EB3)
  M197/1(LL2) -> Eval196/1(In2)
  M197/2(LL3) -> Eval196/2(In3)
  Eval196/1(Out1) -> To Workspace196/1
  [in7] -> M198/1(CT2)
  [in8] -> M198/2(F2)
  [in9] -> M198/3(E2)
  [in11] -> M198/4(T2)
  [in12] -> M198/5(EB2)
  [in13] -> M198/6(CT3)
  [in14] -> M198/7(F3)
  [in15] -> M198/8(E3)
  [in16] -> M198/9(MR3)
  [in17] -> M198/10(T3)
  [in18] -> M198/11(EB3)
  M198/1(LL2) -> Eval197/1(In2)
  M198/2(LL3) -> Eval197/2(In3)
  Eval197/1(Out1) -> To Workspace197/1
  [in7] -> M199/1(CT2)
  [in8] -> M199/2(F2)
  [in9] -> M199/3(E2)
  [in11] -> M199/4(T2)
  [in12] -> M199/5(EB2)
  [in13] -> M199/6(CT3)
  [in14] -> M199/7(F3)
  [in15] -> M199/8(E3)
  [in16] -> M199/9(MR3)
  [in17] -> M199/10(T3)
  [in18] -> M199/11(EB3)
  M199/1(LL2) -> Eval198/1(In2)
  M199/2(LL3) -> Eval198/2(In3)
  Eval198/1(Out1) -> To Workspace198/1
  [in7] -> M200/1(CT2)
  [in8] -> M200/2(F2)
  [in9] -> M200/3(E2)
  [in11] -> M200/4(T2)
  [in12] -> M200/5(EB2)
  [in13] -> M200/6(CT3)
  [in14] -> M200/7(F3)
  [in15] -> M200/8(E3)
  [in16] -> M200/9(MR3)
  [in17] -> M200/10(T3)
  [in18] -> M200/11(EB3)
  M200/1(LL2) -> Eval199/1(In2)
  M200/2(LL3) -> Eval199/2(In3)
  Eval199/1(Out1) -> To Workspace199/1
  [in7] -> M201/1(CT2)
  [in8] -> M201/2(F2)
  [in9] -> M201/3(E2)
  [in11] -> M201/4(T2)
  [in12] -> M201/5(EB2)
  [in13] -> M201/6(CT3)
  [in14] -> M201/7(F3)
  [in15] -> M201/8(E3)
  [in16] -> M201/9(MR3)
  [in17] -> M201/10(T3)
  [in18] -> M201/11(EB3)
  M201/1(LL2) -> Eval200/1(In2)
  M201/2(LL3) -> Eval200/2(In3)
  Eval200/1(Out1) -> To Workspace200/1
  [in7] -> M202/1(CT2)
  [in8] -> M202/2(F2)
  [in9] -> M202/3(E2)
  [in11] -> M202/4(T2)
  [in12] -> M202/5(EB2)
  [in13] -> M202/6(CT3)
  [in14] -> M202/7(F3)
  [in15] -> M202/8(E3)
  [in16] -> M202/9(MR3)
  [in17] -> M202/10(T3)
  [in18] -> M202/11(EB3)
  M202/1(LL2) -> Eval201/1(In2)
  M202/2(LL3) -> Eval201/2(In3)
  Eval201/1(Out1) -> To Workspace201/1
  [in7] -> M203/1(CT2)
  [in8] -> M203/2(F2)
  [in9] -> M203/3(E2)
  [in11] -> M203/4(T2)
  [in12] -> M203/5(EB2)
  [in13] -> M203/6(CT3)
  [in14] -> M203/7(F3)
  [in15] -> M203/8(E3)
  [in16] -> M203/9(MR3)
  [in17] -> M203/10(T3)
  [in18] -> M203/11(EB3)
  M203/1(LL2) -> Eval202/1(In2)
  M203/2(LL3) -> Eval202/2(In3)
  Eval202/1(Out1) -> To Workspace202/1
  [in7] -> M204/1(CT2)
  [in8] -> M204/2(F2)
  [in9] -> M204/3(E2)
  [in11] -> M204/4(T2)
  [in12] -> M204/5(EB2)
  [in13] -> M204/6(CT3)
  [in14] -> M204/7(F3)
  [in15] -> M204/8(E3)
  [in16] -> M204/9(MR3)
  [in17] -> M204/10(T3)
  [in18] -> M204/11(EB3)
  M204/1(LL2) -> Eval203/1(In2)
  M204/2(LL3) -> Eval203/2(In3)
  Eval203/1(Out1) -> To Workspace203/1
  [in7] -> M205/1(CT2)
  [in8] -> M205/2(F2)
  [in9] -> M205/3(E2)
  [in11] -> M205/4(T2)
  [in12] -> M205/5(EB2)
  [in13] -> M205/6(CT3)
  [in14] -> M205/7(F3)
  [in15] -> M205/8(E3)
  [in16] -> M205/9(MR3)
  [in17] -> M205/10(T3)
  [in18] -> M205/11(EB3)
  M205/1(LL2) -> Eval204/1(In2)
  M205/2(LL3) -> Eval204/2(In3)
  Eval204/1(Out1) -> To Workspace204/1
  [in7] -> M206/1(CT2)
  [in8] -> M206/2(F2)
  [in9] -> M206/3(E2)
  [in11] -> M206/4(T2)
  [in12] -> M206/5(EB2)
  [in13] -> M206/6(CT3)
  [in14] -> M206/7(F3)
  [in15] -> M206/8(E3)
  [in16] -> M206/9(MR3)
  [in17] -> M206/10(T3)
  [in18] -> M206/11(EB3)
  M206/1(LL2) -> Eval205/1(In2)
  M206/2(LL3) -> Eval205/2(In3)
  Eval205/1(Out1) -> To Workspace205/1
  [in7] -> M207/1(CT2)
  [in8] -> M207/2(F2)
  [in9] -> M207/3(E2)
  [in11] -> M207/4(T2)
  [in12] -> M207/5(EB2)
  [in13] -> M207/6(CT3)
  [in14] -> M207/7(F3)
  [in15] -> M207/8(E3)
  [in16] -> M207/9(MR3)
  [in17] -> M207/10(T3)
  [in18] -> M207/11(EB3)
  M207/1(LL2) -> Eval206/1(In2)
  M207/2(LL3) -> Eval206/2(In3)
  Eval206/1(Out1) -> To Workspace206/1
  [in7] -> M208/1(CT2)
  [in8] -> M208/2(F2)
  [in9] -> M208/3(E2)
  [in11] -> M208/4(T2)
  [in12] -> M208/5(EB2)
  [in13] -> M208/6(CT3)
  [in14] -> M208/7(F3)
  [in15] -> M208/8(E3)
  [in16] -> M208/9(MR3)
  [in17] -> M208/10(T3)
  [in18] -> M208/11(EB3)
  M208/1(LL2) -> Eval207/1(In2)
  M208/2(LL3) -> Eval207/2(In3)
  Eval207/1(Out1) -> To Workspace207/1
  [in7] -> M209/1(CT2)
  [in8] -> M209/2(F2)
  [in9] -> M209/3(E2)
  [in11] -> M209/4(T2)
  [in12] -> M209/5(EB2)
  [in13] -> M209/6(CT3)
  [in14] -> M209/7(F3)
  [in15] -> M209/8(E3)
  [in16] -> M209/9(MR3)
  [in17] -> M209/10(T3)
  [in18] -> M209/11(EB3)
  M209/1(LL2) -> Eval208/1(In2)
  M209/2(LL3) -> Eval208/2(In3)
  Eval208/1(Out1) -> To Workspace208/1
  [in7] -> M210/1(CT2)
  [in8] -> M210/2(F2)
  [in9] -> M210/3(E2)
  [in11] -> M210/4(T2)
  [in12] -> M210/5(EB2)
  [in13] -> M210/6(CT3)
  [in14] -> M210/7(F3)
  [in15] -> M210/8(E3)
  [in16] -> M210/9(MR3)
  [in17] -> M210/10(T3)
  [in18] -> M210/11(EB3)
  M210/1(LL2) -> Eval209/1(In2)
  M210/2(LL3) -> Eval209/2(In3)
  Eval209/1(Out1) -> To Workspace209/1
  [in7] -> M211/1(CT2)
  [in8] -> M211/2(F2)
  [in9] -> M211/3(E2)
  [in11] -> M211/4(T2)
  [in12] -> M211/5(EB2)
  [in13] -> M211/6(CT3)
  [in14] -> M211/7(F3)
  [in15] -> M211/8(E3)
  [in16] -> M211/9(MR3)
  [in17] -> M211/10(T3)
  [in18] -> M211/11(EB3)
  M211/1(LL2) -> Eval210/1(In2)
  M211/2(LL3) -> Eval210/2(In3)
  Eval210/1(Out1) -> To Workspace210/1
  [in7] -> M212/1(CT2)
  [in8] -> M212/2(F2)
  [in9] -> M212/3(E2)
  [in11] -> M212/4(T2)
  [in12] -> M212/5(EB2)
  [in13] -> M212/6(CT3)
  [in14] -> M212/7(F3)
  [in15] -> M212/8(E3)
  [in16] -> M212/9(MR3)
  [in17] -> M212/10(T3)
  [in18] -> M212/11(EB3)
  M212/1(LL2) -> Eval211/1(In2)
  M212/2(LL3) -> Eval211/2(In3)
  Eval211/1(Out1) -> To Workspace211/1
  [in7] -> M213/1(CT2)
  [in8] -> M213/2(F2)
  [in9] -> M213/3(E2)
  [in11] -> M213/4(T2)
  [in12] -> M213/5(EB2)
  [in13] -> M213/6(CT3)
  [in14] -> M213/7(F3)
  [in15] -> M213/8(E3)
  [in16] -> M213/9(MR3)
  [in17] -> M213/10(T3)
  [in18] -> M213/11(EB3)
  M213/1(LL2) -> Eval212/1(In2)
  M213/2(LL3) -> Eval212/2(In3)
  Eval212/1(Out1) -> To Workspace212/1
  [in7] -> M214/1(CT2)
  [in8] -> M214/2(F2)
  [in9] -> M214/3(E2)
  [in11] -> M214/4(T2)
  [in12] -> M214/5(EB2)
  [in13] -> M214/6(CT3)
  [in14] -> M214/7(F3)
  [in15] -> M214/8(E3)
  [in16] -> M214/9(MR3)
  [in17] -> M214/10(T3)
  [in18] -> M214/11(EB3)
  M214/1(LL2) -> Eval213/1(In2)
  M214/2(LL3) -> Eval213/2(In3)
  Eval213/1(Out1) -> To Workspace213/1
  [in7] -> M215/1(CT2)
  [in8] -> M215/2(F2)
  [in9] -> M215/3(E2)
  [in11] -> M215/4(T2)
  [in12] -> M215/5(EB2)
  [in13] -> M215/6(CT3)
  [in14] -> M215/7(F3)
  [in15] -> M215/8(E3)
  [in16] -> M215/9(MR3)
  [in17] -> M215/10(T3)
  [in18] -> M215/11(EB3)
  M215/1(LL2) -> Eval214/1(In2)
  M215/2(LL3) -> Eval214/2(In3)
  Eval214/1(Out1) -> To Workspace214/1
  [in7] -> M216/1(CT2)
  [in8] -> M216/2(F2)
  [in9] -> M216/3(E2)
  [in11] -> M216/4(T2)
  [in12] -> M216/5(EB2)
  [in13] -> M216/6(CT3)
  [in14] -> M216/7(F3)
  [in15] -> M216/8(E3)
  [in16] -> M216/9(MR3)
  [in17] -> M216/10(T3)
  [in18] -> M216/11(EB3)
  M216/1(LL2) -> Eval215/1(In2)
  M216/2(LL3) -> Eval215/2(In3)
  Eval215/1(Out1) -> To Workspace215/1
  [in7] -> M217/1(CT2)
  [in8] -> M217/2(F2)
  [in9] -> M217/3(E2)
  [in11] -> M217/4(T2)
  [in12] -> M217/5(EB2)
  [in13] -> M217/6(CT3)
  [in14] -> M217/7(F3)
  [in15] -> M217/8(E3)
  [in16] -> M217/9(MR3)
  [in17] -> M217/10(T3)
  [in18] -> M217/11(EB3)
  M217/1(LL2) -> Eval216/1(In2)
  M217/2(LL3) -> Eval216/2(In3)
  Eval216/1(Out1) -> To Workspace216/1
  [in7] -> M218/1(CT2)
  [in8] -> M218/2(F2)
  [in9] -> M218/3(E2)
  [in11] -> M218/4(T2)
  [in12] -> M218/5(EB2)
  [in13] -> M218/6(CT3)
  [in14] -> M218/7(F3)
  [in15] -> M218/8(E3)
  [in16] -> M218/9(MR3)
  [in17] -> M218/10(T3)
  [in18] -> M218/11(EB3)
  M218/1(LL2) -> Eval217/1(In2)
  M218/2(LL3) -> Eval217/2(In3)
  Eval217/1(Out1) -> To Workspace217/1
  [in7] -> M219/1(CT2)
  [in8] -> M219/2(F2)
  [in9] -> M219/3(E2)
  [in11] -> M219/4(T2)
  [in12] -> M219/5(EB2)
  [in13] -> M219/6(CT3)
  [in14] -> M219/7(F3)
  [in15] -> M219/8(E3)
  [in16] -> M219/9(MR3)
  [in17] -> M219/10(T3)
  [in18] -> M219/11(EB3)
  M219/1(LL2) -> Eval218/1(In2)
  M219/2(LL3) -> Eval218/2(In3)
  Eval218/1(Out1) -> To Workspace218/1
  [in7] -> M220/1(CT2)
  [in8] -> M220/2(F2)
  [in9] -> M220/3(E2)
  [in11] -> M220/4(T2)
  [in12] -> M220/5(EB2)
  [in13] -> M220/6(CT3)
  [in14] -> M220/7(F3)
  [in15] -> M220/8(E3)
  [in16] -> M220/9(MR3)
  [in17] -> M220/10(T3)
  [in18] -> M220/11(EB3)
  M220/1(LL2) -> Eval219/1(In2)
  M220/2(LL3) -> Eval219/2(In3)
  Eval219/1(Out1) -> To Workspace219/1
  [in7] -> M222/1(CT2)
  [in8] -> M222/2(F2)
  [in9] -> M222/3(E2)
  [in11] -> M222/4(T2)
  [in12] -> M222/5(EB2)
  [in13] -> M222/6(CT3)
  [in14] -> M222/7(F3)
  [in15] -> M222/8(E3)
  [in16] -> M222/9(MR3)
  [in17] -> M222/10(T3)
  [in18] -> M222/11(EB3)
  M222/1(LL2) -> Eval221/1(In2)
  M222/2(LL3) -> Eval221/2(In3)
  Eval221/1(Out1) -> To Workspace221/1
  [in7] -> M223/1(CT2)
  [in8] -> M223/2(F2)
  [in9] -> M223/3(E2)
  [in11] -> M223/4(T2)
  [in12] -> M223/5(EB2)
  [in13] -> M223/6(CT3)
  [in14] -> M223/7(F3)
  [in15] -> M223/8(E3)
  [in16] -> M223/9(MR3)
  [in17] -> M223/10(T3)
  [in18] -> M223/11(EB3)
  M223/1(LL2) -> Eval222/1(In2)
  M223/2(LL3) -> Eval222/2(In3)
  Eval222/1(Out1) -> To Workspace222/1
  [in7] -> M224/1(CT2)
  [in8] -> M224/2(F2)
  [in9] -> M224/3(E2)
  [in11] -> M224/4(T2)
  [in12] -> M224/5(EB2)
  [in13] -> M224/6(CT3)
  [in14] -> M224/7(F3)
  [in15] -> M224/8(E3)
  [in16] -> M224/9(MR3)
  [in17] -> M224/10(T3)
  [in18] -> M224/11(EB3)
  M224/1(LL2) -> Eval223/1(In2)
  M224/2(LL3) -> Eval223/2(In3)
  Eval223/1(Out1) -> To Workspace223/1
  [in7] -> M225/1(CT2)
  [in8] -> M225/2(F2)
  [in9] -> M225/3(E2)
  [in11] -> M225/4(T2)
  [in12] -> M225/5(EB2)
  [in13] -> M225/6(CT3)
  [in14] -> M225/7(F3)
  [in15] -> M225/8(E3)
  [in16] -> M225/9(MR3)
  [in17] -> M225/10(T3)
  [in18] -> M225/11(EB3)
  M225/1(LL2) -> Eval224/1(In2)
  M225/2(LL3) -> Eval224/2(In3)
  Eval224/1(Out1) -> To Workspace224/1
  [in7] -> M226/1(CT2)
  [in8] -> M226/2(F2)
  [in9] -> M226/3(E2)
  [in11] -> M226/4(T2)
  [in12] -> M226/5(EB2)
  [in13] -> M226/6(CT3)
  [in14] -> M226/7(F3)
  [in15] -> M226/8(E3)
  [in16] -> M226/9(MR3)
  [in17] -> M226/10(T3)
  [in18] -> M226/11(EB3)
  M226/1(LL2) -> Eval225/1(In2)
  M226/2(LL3) -> Eval225/2(In3)
  Eval225/1(Out1) -> To Workspace225/1
  [in7] -> M227/1(CT2)
  [in8] -> M227/2(F2)
  [in9] -> M227/3(E2)
  [in11] -> M227/4(T2)
  [in12] -> M227/5(EB2)
  [in13] -> M227/6(CT3)
  [in14] -> M227/7(F3)
  [in15] -> M227/8(E3)
  [in16] -> M227/9(MR3)
  [in17] -> M227/10(T3)
  [in18] -> M227/11(EB3)
  M227/1(LL2) -> Eval226/1(In2)
  M227/2(LL3) -> Eval226/2(In3)
  Eval226/1(Out1) -> To Workspace226/1
  [in7] -> M228/1(CT2)
  [in8] -> M228/2(F2)
  [in9] -> M228/3(E2)
  [in11] -> M228/4(T2)
  [in12] -> M228/5(EB2)
  [in13] -> M228/6(CT3)
  [in14] -> M228/7(F3)
  [in15] -> M228/8(E3)
  [in16] -> M228/9(MR3)
  [in17] -> M228/10(T3)
  [in18] -> M228/11(EB3)
  M228/1(LL2) -> Eval227/1(In2)
  M228/2(LL3) -> Eval227/2(In3)
  Eval227/1(Out1) -> To Workspace227/1
  [in7] -> M229/1(CT2)
  [in8] -> M229/2(F2)
  [in9] -> M229/3(E2)
  [in11] -> M229/4(T2)
  [in12] -> M229/5(EB2)
  [in13] -> M229/6(CT3)
  [in14] -> M229/7(F3)
  [in15] -> M229/8(E3)
  [in16] -> M229/9(MR3)
  [in17] -> M229/10(T3)
  [in18] -> M229/11(EB3)
  M229/1(LL2) -> Eval228/1(In2)
  M229/2(LL3) -> Eval228/2(In3)
  Eval228/1(Out1) -> To Workspace228/1
  [in7] -> M230/1(CT2)
  [in8] -> M230/2(F2)
  [in9] -> M230/3(E2)
  [in11] -> M230/4(T2)
  [in12] -> M230/5(EB2)
  [in13] -> M230/6(CT3)
  [in14] -> M230/7(F3)
  [in15] -> M230/8(E3)
  [in16] -> M230/9(MR3)
  [in17] -> M230/10(T3)
  [in18] -> M230/11(EB3)
  M230/1(LL2) -> Eval229/1(In2)
  M230/2(LL3) -> Eval229/2(In3)
  Eval229/1(Out1) -> To Workspace229/1
  [in7] -> M231/1(CT2)
  [in8] -> M231/2(F2)
  [in9] -> M231/3(E2)
  [in11] -> M231/4(T2)
  [in12] -> M231/5(EB2)
  [in13] -> M231/6(CT3)
  [in14] -> M231/7(F3)
  [in15] -> M231/8(E3)
  [in16] -> M231/9(MR3)
  [in17] -> M231/10(T3)
  [in18] -> M231/11(EB3)
  M231/1(LL2) -> Eval230/1(In2)
  M231/2(LL3) -> Eval230/2(In3)
  Eval230/1(Out1) -> To Workspace230/1
  [in7] -> M232/1(CT2)
  [in8] -> M232/2(F2)
  [in9] -> M232/3(E2)
  [in11] -> M232/4(T2)
  [in12] -> M232/5(EB2)
  [in13] -> M232/6(CT3)
  [in14] -> M232/7(F3)
  [in15] -> M232/8(E3)
  [in16] -> M232/9(MR3)
  [in17] -> M232/10(T3)
  [in18] -> M232/11(EB3)
  M232/1(LL2) -> Eval231/1(In2)
  M232/2(LL3) -> Eval231/2(In3)
  Eval231/1(Out1) -> To Workspace231/1
  [in7] -> M233/1(CT2)
  [in8] -> M233/2(F2)
  [in9] -> M233/3(E2)
  [in11] -> M233/4(T2)
  [in12] -> M233/5(EB2)
  [in13] -> M233/6(CT3)
  [in14] -> M233/7(F3)
  [in15] -> M233/8(E3)
  [in16] -> M233/9(MR3)
  [in17] -> M233/10(T3)
  [in18] -> M233/11(EB3)
  M233/1(LL2) -> Eval232/1(In2)
  M233/2(LL3) -> Eval232/2(In3)
  Eval232/1(Out1) -> To Workspace232/1
  [in7] -> M234/1(CT2)
  [in8] -> M234/2(F2)
  [in9] -> M234/3(E2)
  [in11] -> M234/4(T2)
  [in12] -> M234/5(EB2)
  [in13] -> M234/6(CT3)
  [in14] -> M234/7(F3)
  [in15] -> M234/8(E3)
  [in16] -> M234/9(MR3)
  [in17] -> M234/10(T3)
  [in18] -> M234/11(EB3)
  M234/1(LL2) -> Eval233/1(In2)
  M234/2(LL3) -> Eval233/2(In3)
  Eval233/1(Out1) -> To Workspace233/1
  [in7] -> M235/1(CT2)
  [in8] -> M235/2(F2)
  [in9] -> M235/3(E2)
  [in11] -> M235/4(T2)
  [in12] -> M235/5(EB2)
  [in13] -> M235/6(CT3)
  [in14] -> M235/7(F3)
  [in15] -> M235/8(E3)
  [in16] -> M235/9(MR3)
  [in17] -> M235/10(T3)
  [in18] -> M235/11(EB3)
  M235/1(LL2) -> Eval234/1(In2)
  M235/2(LL3) -> Eval234/2(In3)
  Eval234/1(Out1) -> To Workspace234/1
  [in7] -> M236/1(CT2)
  [in8] -> M236/2(F2)
  [in9] -> M236/3(E2)
  [in11] -> M236/4(T2)
  [in12] -> M236/5(EB2)
  [in13] -> M236/6(CT3)
  [in14] -> M236/7(F3)
  [in15] -> M236/8(E3)
  [in16] -> M236/9(MR3)
  [in17] -> M236/10(T3)
  [in18] -> M236/11(EB3)
  M236/1(LL2) -> Eval235/1(In2)
  M236/2(LL3) -> Eval235/2(In3)
  Eval235/1(Out1) -> To Workspace235/1
  [in7] -> M237/1(CT2)
  [in8] -> M237/2(F2)
  [in9] -> M237/3(E2)
  [in11] -> M237/4(T2)
  [in12] -> M237/5(EB2)
  [in13] -> M237/6(CT3)
  [in14] -> M237/7(F3)
  [in15] -> M237/8(E3)
  [in16] -> M237/9(MR3)
  [in17] -> M237/10(T3)
  [in18] -> M237/11(EB3)
  M237/1(LL2) -> Eval236/1(In2)
  M237/2(LL3) -> Eval236/2(In3)
  Eval236/1(Out1) -> To Workspace236/1
  [in7] -> M238/1(CT2)
  [in8] -> M238/2(F2)
  [in9] -> M238/3(E2)
  [in11] -> M238/4(T2)
  [in12] -> M238/5(EB2)
  [in13] -> M238/6(CT3)
  [in14] -> M238/7(F3)
  [in15] -> M238/8(E3)
  [in16] -> M238/9(MR3)
  [in17] -> M238/10(T3)
  [in18] -> M238/11(EB3)
  M238/1(LL2) -> Eval237/1(In2)
  M238/2(LL3) -> Eval237/2(In3)
  Eval237/1(Out1) -> To Workspace237/1
  [in7] -> M239/1(CT2)
  [in8] -> M239/2(F2)
  [in9] -> M239/3(E2)
  [in11] -> M239/4(T2)
  [in12] -> M239/5(EB2)
  [in13] -> M239/6(CT3)
  [in14] -> M239/7(F3)
  [in15] -> M239/8(E3)
  [in16] -> M239/9(MR3)
  [in17] -> M239/10(T3)
  [in18] -> M239/11(EB3)
  M239/1(LL2) -> Eval238/1(In2)
  M239/2(LL3) -> Eval238/2(In3)
  Eval238/1(Out1) -> To Workspace238/1
  [in7] -> M240/1(CT2)
  [in8] -> M240/2(F2)
  [in9] -> M240/3(E2)
  [in11] -> M240/4(T2)
  [in12] -> M240/5(EB2)
  [in13] -> M240/6(CT3)
  [in14] -> M240/7(F3)
  [in15] -> M240/8(E3)
  [in16] -> M240/9(MR3)
  [in17] -> M240/10(T3)
  [in18] -> M240/11(EB3)
  M240/1(LL2) -> Eval239/1(In2)
  M240/2(LL3) -> Eval239/2(In3)
  Eval239/1(Out1) -> To Workspace239/1
  [in7] -> M241/1(CT2)
  [in8] -> M241/2(F2)
  [in9] -> M241/3(E2)
  [in11] -> M241/4(T2)
  [in12] -> M241/5(EB2)
  [in13] -> M241/6(CT3)
  [in14] -> M241/7(F3)
  [in15] -> M241/8(E3)
  [in16] -> M241/9(MR3)
  [in17] -> M241/10(T3)
  [in18] -> M241/11(EB3)
  M241/1(LL2) -> Eval240/1(In2)
  M241/2(LL3) -> Eval240/2(In3)
  Eval240/1(Out1) -> To Workspace240/1
  [in7] -> M242/1(CT2)
  [in8] -> M242/2(F2)
  [in9] -> M242/3(E2)
  [in11] -> M242/4(T2)
  [in12] -> M242/5(EB2)
  [in13] -> M242/6(CT3)
  [in14] -> M242/7(F3)
  [in15] -> M242/8(E3)
  [in16] -> M242/9(MR3)
  [in17] -> M242/10(T3)
  [in18] -> M242/11(EB3)
  M242/1(LL2) -> Eval241/1(In2)
  M242/2(LL3) -> Eval241/2(In3)
  Eval241/1(Out1) -> To Workspace241/1
  [in7] -> M243/1(CT2)
  [in8] -> M243/2(F2)
  [in9] -> M243/3(E2)
  [in11] -> M243/4(T2)
  [in12] -> M243/5(EB2)
  [in13] -> M243/6(CT3)
  [in14] -> M243/7(F3)
  [in15] -> M243/8(E3)
  [in16] -> M243/9(MR3)
  [in17] -> M243/10(T3)
  [in18] -> M243/11(EB3)
  M243/1(LL2) -> Eval242/1(In2)
  M243/2(LL3) -> Eval242/2(In3)
  Eval242/1(Out1) -> To Workspace242/1
  [in7] -> M244/1(CT2)
  [in8] -> M244/2(F2)
  [in9] -> M244/3(E2)
  [in11] -> M244/4(T2)
  [in12] -> M244/5(EB2)
  [in13] -> M244/6(CT3)
  [in14] -> M244/7(F3)
  [in15] -> M244/8(E3)
  [in16] -> M244/9(MR3)
  [in17] -> M244/10(T3)
  [in18] -> M244/11(EB3)
  M244/1(LL2) -> Eval243/1(In2)
  M244/2(LL3) -> Eval243/2(In3)
  Eval243/1(Out1) -> To Workspace243/1
  [in7] -> M245/1(CT2)
  [in8] -> M245/2(F2)
  [in9] -> M245/3(E2)
  [in11] -> M245/4(T2)
  [in12] -> M245/5(EB2)
  [in13] -> M245/6(CT3)
  [in14] -> M245/7(F3)
  [in15] -> M245/8(E3)
  [in16] -> M245/9(MR3)
  [in17] -> M245/10(T3)
  [in18] -> M245/11(EB3)
  M245/1(LL2) -> Eval244/1(In2)
  M245/2(LL3) -> Eval244/2(In3)
  Eval244/1(Out1) -> To Workspace244/1
  [in7] -> M246/1(CT2)
  [in8] -> M246/2(F2)
  [in9] -> M246/3(E2)
  [in11] -> M246/4(T2)
  [in12] -> M246/5(EB2)
  [in13] -> M246/6(CT3)
  [in14] -> M246/7(F3)
  [in15] -> M246/8(E3)
  [in16] -> M246/9(MR3)
  [in17] -> M246/10(T3)
  [in18] -> M246/11(EB3)
  M246/1(LL2) -> Eval245/1(In2)
  M246/2(LL3) -> Eval245/2(In3)
  Eval245/1(Out1) -> To Workspace245/1
  Inputs/1(CT2) -> dtc_CT2/1
  dtc_CT2/1 -> CPSUT/1(CT2), [in7]
  Inputs/2(F2) -> dtc_F2/1
  dtc_F2/1 -> CPSUT/2(F2), [in8]
  Inputs/3(E2) -> dtc_E2/1
  dtc_E2/1 -> CPSUT/3(E2), [in9]
  Inputs/4(T2) -> dtc_T2/1
  dtc_T2/1 -> CPSUT/4(T2), [in11]
  Inputs/5(EB2) -> dtc_EB2/1
  dtc_EB2/1 -> CPSUT/5(EB2), [in12]
  Inputs/6(CT3) -> dtc_CT3/1
  dtc_CT3/1 -> CPSUT/6(CT3), [in13]
  Inputs/7(F3) -> dtc_F3/1
  dtc_F3/1 -> CPSUT/7(F3), [in14]
  Inputs/8(E3) -> dtc_E3/1
  dtc_E3/1 -> CPSUT/8(E3), [in15]
  Inputs/9(MR3) -> dtc_MR3/1
  dtc_MR3/1 -> CPSUT/9(MR3), [in16]
  Inputs/10(T3) -> dtc_T3/1
  dtc_T3/1 -> CPSUT/10(T3), [in17]
  Inputs/11(EB3) -> dtc_EB3/1
  dtc_EB3/1 -> CPSUT/11(EB3), [in18]
